simulink model "drop_referance_gen"  (R2025b)
settings: Solver=VariableStepAuto  StartTime=0.0  StopTime=5  FixedStep=1/1000  MaxStep=1e-4  RelTol=1e-3
model workspace (MAT data in the model file):
  h_drop = 3
libraries: simulink x14, eeGeneralControl x6
settings Model: Creator=karadeli  LastModifiedBy=karadeli

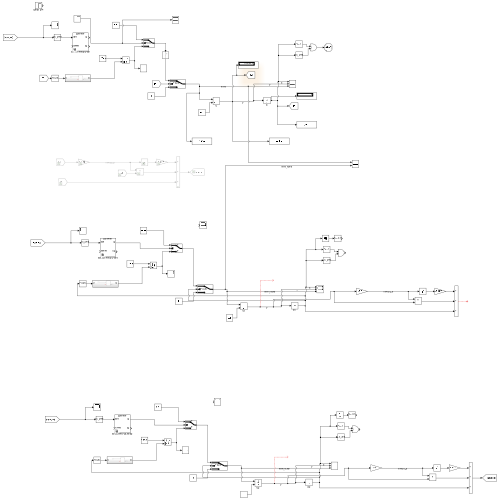
[thumbnail: Simulink's stored preview of the top-level diagram]
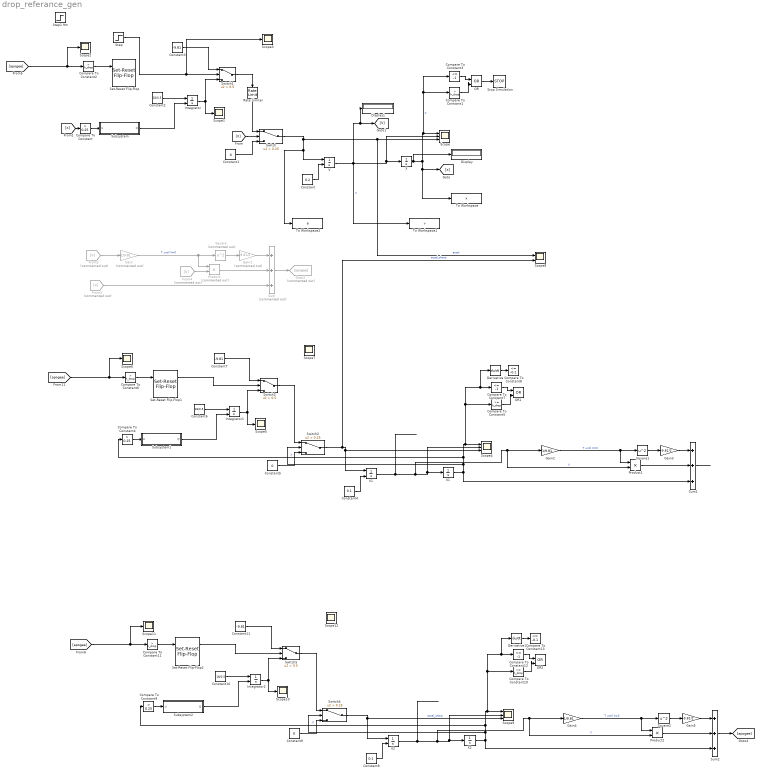
== system drop_referance_gen ==
  Compare To Constant : simulink/Logic and Bit Operations/Compare To Constant  relop=>  const=0.25  OutDataTypeStr=boolean
  Compare To Constant{1..2,6,11} (4 alike) : simulink/Logic and Bit Operations/Compare To Constant  relop=>  const=h_drop  OutDataTypeStr=boolean
  Compare To Constant10 : simulink/Logic and Bit Operations/Compare To Constant  relop=>=  const=h_drop  OutDataTypeStr=boolean
  Compare To Constant12 : simulink/Logic and Bit Operations/Compare To Constant  relop=<=  const=-1  OutDataTypeStr=boolean
  Compare To Constant13 : simulink/Logic and Bit Operations/Compare To Constant  relop=<=  const=-0.1  OutDataTypeStr=boolean
  Compare To Constant3 : simulink/Logic and Bit Operations/Compare To Constant  relop=<=  const=-1  OutDataTypeStr=boolean
  Compare To Constant4 : simulink/Logic and Bit Operations/Compare To Constant  relop=>  const=0.25  OutDataTypeStr=boolean
  Compare To Constant5 : simulink/Logic and Bit Operations/Compare To Constant  relop=>=  const=h_drop  OutDataTypeStr=boolean
  Compare To Constant7 : simulink/Logic and Bit Operations/Compare To Constant  relop=<=  const=-1  OutDataTypeStr=boolean
  Compare To Constant8 : simulink/Logic and Bit Operations/Compare To Constant  relop=<=  const=-0.1  OutDataTypeStr=boolean
  Compare To Constant9 : simulink/Logic and Bit Operations/Compare To Constant  relop=>  const=0.25  OutDataTypeStr=boolean
  Constant : Constant  Value=0.2
  Constant1 : Constant  Value=0
  Constant10 : Constant  Value=18/0.5
  Constant11 : Constant  Value=-9.81
  Constant2 : Constant  Value=18/0.5
  Constant3 : Constant  Value=-9.81
  Constant4 : Constant  Value=0.1
  Constant5 : Constant  Value=0
  Constant6 : Constant  Value=18/0.5
  Constant7 : Constant  Value=-9.81
  Constant8 : Constant  Value=0.1
  Constant9 : Constant  Value=0
  Derivative : Derivative
  Derivative1 : Derivative
  Display : Display
  Display1 : Display
  From2 : From  Commented=on  GotoTag=V
  From3 : From  Commented=on  GotoTag=X
  From4 : From  Commented=on  GotoTag=V
  Gain : Gain  Commented=on  Gain=1/9.81
  Gain1 : Gain  Commented=on  Gain=-9.81/2
  Gain2 : Gain  Gain=1/9.81
  Gain3 : Gain  Gain=-9.81/2
  Gain4 : Gain  Gain=1/9.81
  Gain5 : Gain  Gain=-9.81/2
  Goto2 : Goto  Commented=on  GotoTag=apogee
  Integrator : Integrator  ExternalReset=level  LimitOutput=on  UpperSaturationLimit=18  LowerSaturationLimit=0
  Integrator1 : Integrator  ExternalReset=level  LimitOutput=on  UpperSaturationLimit=18  LowerSaturationLimit=0
  Integrator2 : Integrator  ExternalReset=level  LimitOutput=on  UpperSaturationLimit=18  LowerSaturationLimit=0
  OR : Logic  Operator=OR  IconShape=distinctive  AllPortsSameDT=off  OutDataTypeStr=boolean
  OR1 : Logic  Operator=OR  IconShape=distinctive  AllPortsSameDT=off  OutDataTypeStr=boolean
  OR2 : Logic  Operator=OR  IconShape=distinctive  AllPortsSameDT=off  OutDataTypeStr=boolean
  Product : Product  Commented=on
  Product1 : Product
  Product2 : Product
  Rate Limiter : RateLimiter  RisingSlewLimit=(18+9.81)/0.3  FallingSlewLimit=-(18+9.81)/0.3  SampleTimeMode=inherited
  Scope : Scope  NumInputPorts=3
      settings: ActiveDisplayYMinimum=-0.37499963638695161  ActiveDisplayYMaximum=3.3749967274825652
  Scope{1..3,5..7,10..12} (9 alike) : Scope
      Scope1 settings: ActiveDisplayYMinimum=-2.2499999999999996  ActiveDisplayYMaximum=20.25
      Scope10 settings: ActiveDisplayYMinimum=-2.2499999999999996  ActiveDisplayYMaximum=20.25  DataLoggingVariableName=ScopeData9
      Scope11 settings: ActiveDisplayYMinimum=-40.104603035926139  ActiveDisplayYMaximum=17.886239672819958  DataLoggingVariableName=ScopeData10
      Scope12 settings: ActiveDisplayYMinimum=-0.12499999999999997  ActiveDisplayYMaximum=1.125  DataLoggingVariableName=ScopeData11
      Scope2 settings: ActiveDisplayYMinimum=-40.104603035926139  ActiveDisplayYMaximum=17.886239672819958  DataLoggingVariableName=ScopeData2
      Scope3 settings: ActiveDisplayYMinimum=-0.12499999999999997  ActiveDisplayYMaximum=1.125  DataLoggingVariableName=ScopeData3
      Scope5 settings: ActiveDisplayYMinimum=-2.2499999999999996  ActiveDisplayYMaximum=20.25  DataLoggingVariableName=ScopeData5
      Scope6 settings: ActiveDisplayYMinimum=-40.104603035926139  ActiveDisplayYMaximum=17.886239672819958  DataLoggingVariableName=ScopeData6
      Scope7 settings: ActiveDisplayYMinimum=-0.12499999999999997  ActiveDisplayYMaximum=1.125  DataLoggingVariableName=ScopeData7
  Scope4 : Scope  NumInputPorts=3
      settings: ActiveDisplayYMinimum=-0.62499999994592126  ActiveDisplayYMaximum=5.6249999995132924  DataLoggingVariableName=ScopeData4
  Scope8 : Scope  NumInputPorts=2
      settings: ActiveDisplayYMinimum=-13.28625  ActiveDisplayYMaximum=21.47625  DataLoggingVariableName=ScopeData8
  Scope9 : Scope  NumInputPorts=3
      settings: ActiveDisplayYMinimum=-0.62499999994592126  ActiveDisplayYMaximum=5.6249999995132924  DataLoggingVariableName=ScopeData12
  Set-Reset Flip-Flop : eeGeneralControl/Set-Reset Flip-Flop  LabelModeActiveChoice=Discrete  UndefState=Set  Q0=0  Ts=-1
      settings: LibrarySourceBlock=ee_sl_lib/General Control/Set-Reset Flip-Flop
  Set-Reset Flip-Flop1 : eeGeneralControl/Set-Reset Flip-Flop  LabelModeActiveChoice=Discrete  UndefState=Set  Q0=0  Ts=-1
      settings: LibrarySourceBlock=ee_sl_lib/General Control/Set-Reset Flip-Flop
  Set-Reset Flip-Flop2 : eeGeneralControl/Set-Reset Flip-Flop  LabelModeActiveChoice=Discrete  UndefState=Set  Q0=0  Ts=-1
      settings: LibrarySourceBlock=ee_sl_lib/General Control/Set-Reset Flip-Flop
  Square : Math  Commented=on  Operator=square
  Square1 : Math  Operator=square
  Square2 : Math  Operator=square
  Step : Step  Time=1.6809355  SampleTime=0
  Step1 9m : Step  Time=3.1764425222  SampleTime=0
  Stop Simulation : Stop
  Subsystem : Subsystem
  Subsystem1 : Subsystem
  Subsystem2 : Subsystem
  Sum : Sum  Commented=on  Inputs=+++
  Sum1 : Sum  Inputs=+++
  Sum2 : Sum  Inputs=+++
  Switch : Switch  Criteria=u2 > Threshold  Threshold=0.25  SaturateOnIntegerOverflow=off  InputSameDT=off
  Switch1 : Switch  Criteria=u2 > Threshold  Threshold=0.5  SaturateOnIntegerOverflow=off  InputSameDT=off
  Switch2 : Switch  Criteria=u2 > Threshold  Threshold=0.25  SaturateOnIntegerOverflow=off  InputSameDT=off
  Switch3 : Switch  Criteria=u2 > Threshold  Threshold=0.5  SaturateOnIntegerOverflow=off  InputSameDT=off
  Switch4 : Switch  Criteria=u2 > Threshold  Threshold=0.25  SaturateOnIntegerOverflow=off  InputSameDT=off
  Switch5 : Switch  Criteria=u2 > Threshold  Threshold=0.5  SaturateOnIntegerOverflow=off  InputSameDT=off
  To Workspace : ToWorkspace  VariableName=x  SaveFormat=Timeseries  SampleTime=-1
  To Workspace1 : ToWorkspace  VariableName=v  SaveFormat=Timeseries  SampleTime=-1
  To Workspace2 : ToWorkspace  VariableName=a  SaveFormat=Timeseries  SampleTime=-1
  V : Integrator  InitialConditionSource=external
  V1 : Integrator  InitialConditionSource=external
  V2 : Integrator  InitialConditionSource=external
  X : Integrator
  X1 : Integrator
  X2 : Integrator
  wires:
  V/1 -> Display1/1, [V], To Workspace1/1, Scope/2, X/1  "V"
  X/1 -> Display/1, Compare To Constant3/1, Compare To Constant1/1, Scope/1, To Workspace/1, [X]  "X"
  Constant/1 -> V/2
  [X] -> Switch/2
  Constant1/1 -> Switch/3
  Switch/1 -> To Workspace2/1, V/1, Scope8/1, Scope/3  "accel"
  [X] -> Compare To Constant/1
  Compare To Constant/1 -> Subsystem/1(U)
  Subsystem/1(Q) -> Integrator/2
  Constant2/1 -> Integrator/1
  Integrator/1 -> Scope1/1, Switch1/3
  From2/1 -> Gain/1
  Gain/1 -> Product/1, Square/1  "T until V=0"
  Square/1 -> Gain1/1
  Gain1/1 -> Sum/1
  From3/1 -> Sum/3
  From4/1 -> Product/2
  Product/1 -> Sum/2
  Sum/1 -> Goto2/1
  Constant3/1 -> Switch1/1
  Switch1/1 -> Rate Limiter/1
  Compare To Constant1/1 -> OR/2
  Step/1 -> Scope3/1, Switch1/2
  Compare To Constant2/1 -> Set-Reset Flip-Flop/1
  Compare To Constant3/1 -> OR/1
  [apogee] -> Scope2/1, Compare To Constant2/1
  Rate Limiter/1 -> Switch/1
  Constant4/1 -> V1/2
  Compare To Constant5/1 -> OR1/2
  X1/1 -> Switch2/2, Compare To Constant4/1, Derivative/1, Compare To Constant7/1, Compare To Constant5/1, Scope4/1, Sum1/3  "X"
  Compare To Constant6/1 -> Set-Reset Flip-Flop1/1
  [apogee] -> Scope6/1, Compare To Constant6/1
  Switch2/1 -> Scope8/2, V1/1, Scope4/3  "accel_sharp"
  Compare To Constant7/1 -> OR1/1
  Constant7/1 -> Switch3/1
  Constant6/1 -> Integrator1/1
  V1/1 -> Product1/2, Gain2/1, Scope4/2, X1/1  "V"
  Compare To Constant4/1 -> Subsystem1/1(U)
  Constant5/1 -> Switch2/3
  Switch3/1 -> Switch2/1
  Subsystem1/1(Q) -> Integrator1/2
  Integrator1/1 -> Scope5/1, Switch3/3
  Set-Reset Flip-Flop1/1 -> Switch3/2
  Sum1/1 -> ?
  Product1/1 -> Sum1/2
  Gain3/1 -> Sum1/1
  Square1/1 -> Gain3/1
  Gain2/1 -> Square1/1, Product1/1  "T until V=0"
  Derivative/1 -> Compare To Constant8/1
  Derivative1/1 -> Compare To Constant13/1
  Gain4/1 -> Product2/1, Square2/1  "T until V=0"
  Square2/1 -> Gain5/1
  Gain5/1 -> Sum2/1
  Product2/1 -> Sum2/2
  Sum2/1 -> [apogee]
  Set-Reset Flip-Flop2/1 -> Switch5/2
  Integrator2/1 -> Switch5/3, Scope10/1
  Subsystem2/1(Q) -> Integrator2/2
  Switch5/1 -> Switch4/1
  Constant9/1 -> Switch4/3
  Compare To Constant9/1 -> Subsystem2/1(U)
  V2/1 -> X2/1, Scope9/2, Gain4/1, Product2/2  "V"
  Constant10/1 -> Integrator2/1
  Constant11/1 -> Switch5/1
  Compare To Constant12/1 -> OR2/1
  Switch4/1 -> Scope9/3, V2/1  "accel_sharp"
  [apogee] -> Compare To Constant11/1, Scope11/1
  Compare To Constant11/1 -> Set-Reset Flip-Flop2/1
  X2/1 -> Sum2/3, Scope9/1, Compare To Constant10/1, Compare To Constant12/1, Derivative1/1, Compare To Constant9/1, Switch4/2  "X"
  Compare To Constant10/1 -> OR2/2
  Constant8/1 -> V2/2
  OR/1 -> Stop Simulation/1

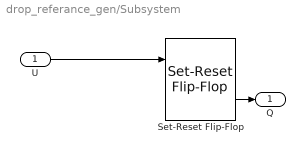
== system drop_referance_gen/Subsystem ==
  U : Inport
  Set-Reset Flip-Flop : eeGeneralControl/Set-Reset Flip-Flop  LabelModeActiveChoice=Discrete  UndefState=Set  Q0=0  Ts=-1
      settings: LibrarySourceBlock=ee_sl_lib/General Control/Set-Reset Flip-Flop
  Q : Outport
  wires:
  Set-Reset Flip-Flop/2 -> Q/1
  ? -> Set-Reset Flip-Flop/2
  U/1 -> Set-Reset Flip-Flop/1

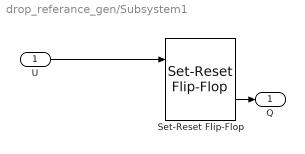
== system drop_referance_gen/Subsystem1 ==
  U : Inport
  Set-Reset Flip-Flop : eeGeneralControl/Set-Reset Flip-Flop  LabelModeActiveChoice=Discrete  UndefState=Set  Q0=0  Ts=-1
      settings: LibrarySourceBlock=ee_sl_lib/General Control/Set-Reset Flip-Flop
  Q : Outport
  wires:
  Set-Reset Flip-Flop/2 -> Q/1
  ? -> Set-Reset Flip-Flop/2
  U/1 -> Set-Reset Flip-Flop/1

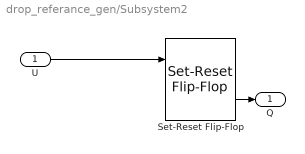
== system drop_referance_gen/Subsystem2 ==
  U : Inport
  Set-Reset Flip-Flop : eeGeneralControl/Set-Reset Flip-Flop  LabelModeActiveChoice=Discrete  UndefState=Set  Q0=0  Ts=-1
      settings: LibrarySourceBlock=ee_sl_lib/General Control/Set-Reset Flip-Flop
  Q : Outport
  wires:
  U/1 -> Set-Reset Flip-Flop/1
  ? -> Set-Reset Flip-Flop/2
  Set-Reset Flip-Flop/2 -> Q/1
